simulink model "PNO_Module_Test"  (R2025a)
settings: Solver=VariableStepAuto  StartTime=0.0  StopTime=10.0  RelTol=1e-3
undefined symbols (not defined in the file): D_delta, D_initial, D_lowerlimit, D_upperlimit
settings Model: Creator=LiHaoh  LastModifiedBy=li_hh

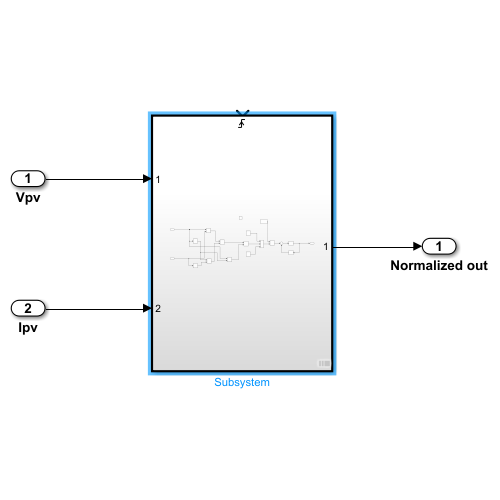
[thumbnail: Simulink's stored preview of the top-level diagram]
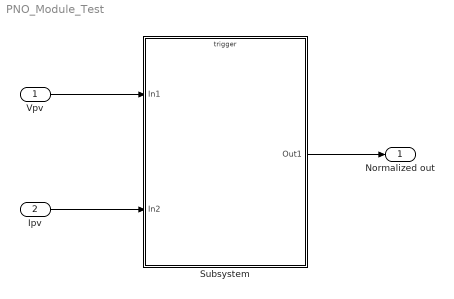
== system PNO_Module_Test ==
  Vpv : Inport
  Ipv : Inport  Port=2
  Subsystem : Subsystem
  Normalized out : Outport
  wires:
  Vpv/1 -> Subsystem/1(In1)
  Ipv/1 -> Subsystem/2(In2)
  Subsystem/1(Out1) -> Normalized out/1

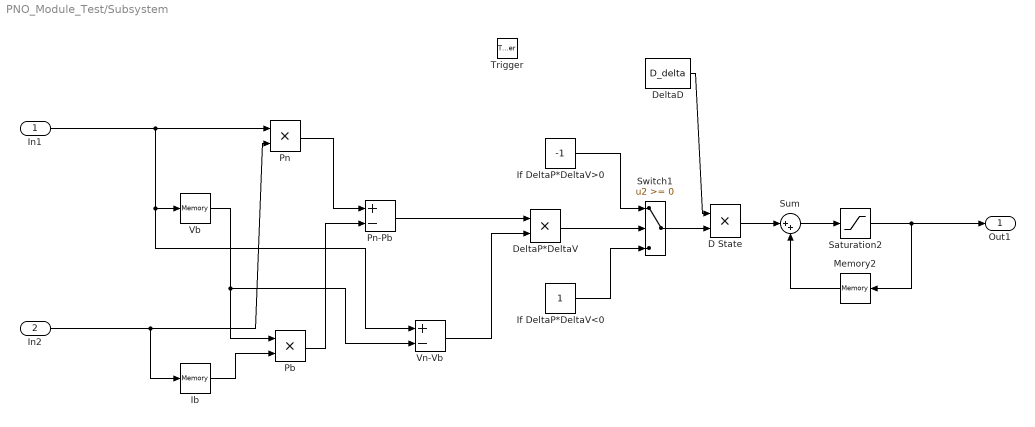
== system PNO_Module_Test/Subsystem ==
  In1 : Inport
  In2 : Inport  Port=2
  Trigger : TriggerPort  VariantControl=(inherit)  PortDimensions=1
  D State : Product  RndMeth=Zero
  DeltaD : Constant  Value=D_delta
  DeltaP*DeltaV : Product  RndMeth=Zero
  Ib : Memory  InheritSampleTime=on  LinearizeAsDelay=on
  If DeltaP*DeltaV<0 : Constant
  If DeltaP*DeltaV>0 : Constant  Value=-1
  Memory2 : Memory  InitialCondition=D_initial  InheritSampleTime=on
  Pb : Product  RndMeth=Zero
  Pn : Product  RndMeth=Zero
  Pn-Pb : Sum  Inputs=+-
  Saturation2 : Saturate  UpperLimit=D_upperlimit  LowerLimit=D_lowerlimit
  Sum : Sum  Inputs=|++
  Switch1 : Switch  SaturateOnIntegerOverflow=off  InputSameDT=off
  Vb : Memory  InheritSampleTime=on  LinearizeAsDelay=on
  Vn-Vb : Sum  Inputs=+-
  Out1 : Outport
  wires:
  If DeltaP*DeltaV>0/1 -> Switch1/1
  Switch1/1 -> D State/2
  Pb/1 -> Pn-Pb/2
  D State/1 -> Sum/1
  Saturation2/1 -> Out1/1, Memory2/1
  If DeltaP*DeltaV<0/1 -> Switch1/3
  Pn/1 -> Pn-Pb/1
  DeltaD/1 -> D State/1
  In1/1 -> Vn-Vb/1, Vb/1, Pn/1
  Vn-Vb/1 -> DeltaP*DeltaV/2
  Ib/1 -> Pb/2
  Sum/1 -> Saturation2/1
  DeltaP*DeltaV/1 -> Switch1/2
  In2/1 -> Pn/2, Ib/1
  Pn-Pb/1 -> DeltaP*DeltaV/1
  Memory2/1 -> Sum/2
  Vb/1 -> Vn-Vb/2, Pb/1
